simulink model "slGTC_3gdl"  (Simulink 9.0)
settings: Solver=ode45  StartTime=0.0  StopTime=Tsim  MaxStep=1e-3  RelTol=1e-8  EnableMultiTasking=on
values from neighbouring files (symbols this model uses):
  duracion = 1    [simulaciones.m]
  n = 5    [simulaciones.m]
  t_ini = 0.5    [simulaciones.m]
  Tm = 0.001    [Controlre.m]    (also in controles.m; simulaciones.m)
  XYZfin = CinematicaDirecta([1 1 1])    [simulaciones.m]
  XYZini = CinematicaDirecta([0 0 0])    [simulaciones.m]
settings Model: Creator=Manuel G. Ortega  LastModifiedBy=Alvaro  ExtModeTrigMode=oneshot  ExtModeArmWhenConnect=off
settings DataIOCC: SignalLoggingSaveFormat=ModelDataLogs
settings OptimizationCC: BooleanDataType=off  ExpressionDepthLimit=2147483647  InitFltsAndDblsToZero=on
settings DebuggingCC: SaveWithParameterizedLinksMsg=none  SignalResolutionControl=TryResolveAllWithWarning  MultiTaskDSMMsg=warning  MultiTaskCondExecSysMsg=none  FcnCallInpInsideContextMsg=warning  StateNameClashWarn=warning  StrictBusMsg=None
settings HardwareCC: TargetUnknown=on
settings GRTTargetCC: TargetFcnLib=ansi_tfl_tmw.mat  GeneratePreprocessorConditionals=Disable all  CombineOutputUpdateFcns=off  GRTInterface=on
settings ConfigComp: CovSFcnEnable=off

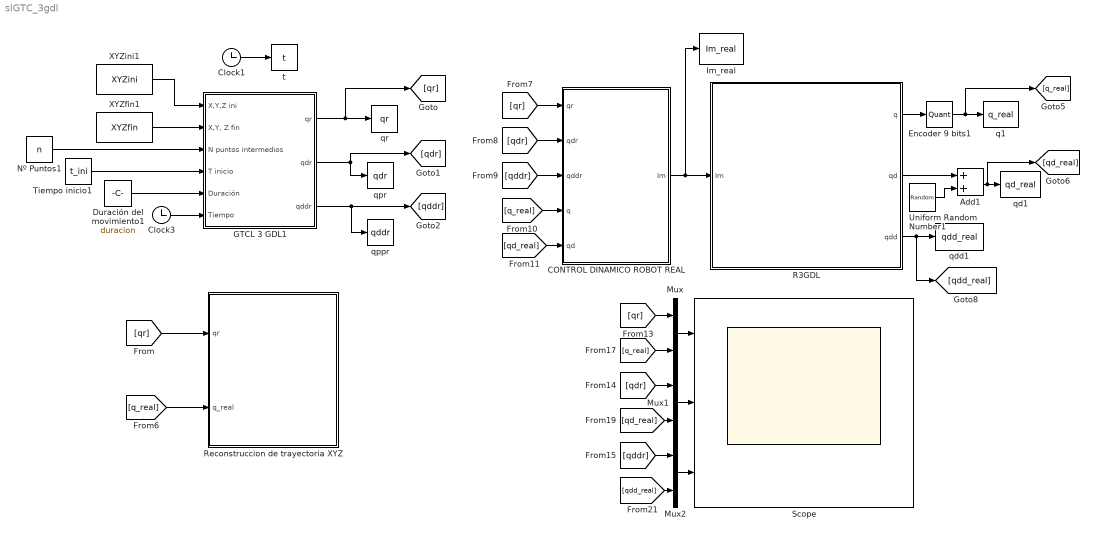
== system slGTC_3gdl ==
  Add1 : Sum
  CONTROL DINAMICO ROBOT REAL : Subsystem
  Clock1 : Clock
  Clock3 : Clock
  Duración del movimiento1 : Constant  Value=duracion
  Encoder 9 bits1 : Quantizer  QuantizationInterval=2*pi/(2^9)
  GTCL 3 GDL1 : Subsystem
  Im_real : ToWorkspace  VariableName=Im_real
  Mux : Mux  Inputs=2
  Mux1 : Mux  Inputs=2
  Mux2 : Mux  Inputs=2
  Nº Puntos1 : Constant  Value=n
  R3GDL : Subsystem  mask(Control y Programación de Robots (4 GIERM)){NGrupo=3, q1_ini=0, q2_ini=0, q3_ini=0, Bl_q1=off, Bl_q2=off, Bl_q3=off, AccionamientoDirecto=on}
      mask prompts: NGrupo "Nº de GRUPO"; q1_ini "q1 inicial  (rad)"; q2_ini "q2 inicial (rad)"; q3_ini "q3_inicial (rad)"; Bl_q1 "Bloqueo q1"; Bl_q2 "Bloqueo q2"; Bl_q3 "Bloqueo q3"; AccionamientoDirecto "Accionamiento directo"
      mask help: Robot de 3 grados de libertad RRR
      mask Display:
      | image(imread('R3GDL_RRR.JPG'));
      | port_label('output', 1, 'q');
      | port_label('output', 2, 'qd');
      | port_label('output', 3, 'qdd');
      | port_label('input', 1, 'Im')
  Reconstruccion de trayectoria XYZ : Subsystem
  Scope : Scope  NumInputPorts=3
  Tiempo inicio1 : Constant  Value=t_ini
  Uniform Random Number1 : UniformRandomNumber  Minimum=-1500*2*pi/60*0.01  Maximum=1500*2*pi/60*0.01  SampleTime=Tm/10
  XYZfin1 : Constant  Value=XYZfin
  XYZini1 : Constant  Value=XYZini
  q1 : ToWorkspace  VariableName=q_real  SampleTime=-1
  qd1 : ToWorkspace  VariableName=qd_real  SampleTime=-1
  qdd1 : ToWorkspace  VariableName=qdd_real  SampleTime=-1
  qppr : ToWorkspace  VariableName=qddr  SampleTime=-1
  qpr : ToWorkspace  VariableName=qdr  SampleTime=-1
  qr : ToWorkspace  VariableName=qr  SampleTime=-1
  t : ToWorkspace  VariableName=t  SampleTime=-1
  wires:
  GTCL 3 GDL1/1(qr) -> [qr], qr/1
  GTCL 3 GDL1/2(qdr) -> qpr/1, [qdr]
  GTCL 3 GDL1/3(qddr) -> qppr/1, [qddr]
  Clock3/1 -> GTCL 3 GDL1/6(Tiempo)
  XYZini1/1 -> GTCL 3 GDL1/1(X,Y,Z ini)
  Clock1/1 -> t/1
  Nº Puntos1/1 -> GTCL 3 GDL1/3(N puntos intermedios)
  Tiempo inicio1/1 -> GTCL 3 GDL1/4(T inicio)
  Duración del movimiento1/1 -> GTCL 3 GDL1/5(Duración)
  XYZfin1/1 -> GTCL 3 GDL1/2("X,Y, Z fin")
  [qd_real] -> CONTROL DINAMICO ROBOT REAL/5(qd)
  [q_real] -> CONTROL DINAMICO ROBOT REAL/4(q)
  [qddr] -> CONTROL DINAMICO ROBOT REAL/3(qddr)
  [qdr] -> CONTROL DINAMICO ROBOT REAL/2(qdr)
  [qr] -> CONTROL DINAMICO ROBOT REAL/1(qr)
  CONTROL DINAMICO ROBOT REAL/1(Im) -> Im_real/1, R3GDL/1(Im)
  R3GDL/3(qdd) -> [qdd_real], qdd1/1
  [qr] -> Reconstruccion de trayectoria XYZ/1(qr)
  [q_real] -> Reconstruccion de trayectoria XYZ/2(q_real)
  Mux/1 -> Scope/1
  Mux1/1 -> Scope/2
  Mux2/1 -> Scope/3
  [qr] -> Mux/1
  [qdr] -> Mux1/1
  [qddr] -> Mux2/1
  [q_real] -> Mux/2
  [qd_real] -> Mux1/2
  [qdd_real] -> Mux2/2
  Uniform Random Number1/1 -> Add1/2
  R3GDL/1(q) -> Encoder 9 bits1/1
  Encoder 9 bits1/1 -> [q_real], q1/1
  R3GDL/2(qd) -> Add1/1
  Add1/1 -> [qd_real], qd1/1

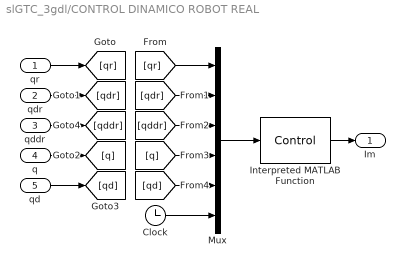
== system slGTC_3gdl/CONTROL DINAMICO ROBOT REAL ==
  qr : Inport
  qdr : Inport  Port=2
  qddr : Inport  Port=3
  q : Inport  Port=4
  qd : Inport  Port=5
  Clock : Clock
  Interpreted MATLAB Function : MATLABFcn  MATLABFcn=Control  SampleTime=Tm
  Mux : Mux  Inputs=6
  Im : Outport
  wires:
  [qddr] -> Mux/3
  [qd] -> Mux/5
  [q] -> Mux/4
  [qr] -> Mux/1
  [qdr] -> Mux/2
  Clock/1 -> Mux/6
  Mux/1 -> Interpreted MATLAB Function/1
  Interpreted MATLAB Function/1 -> Im/1
  qddr/1 -> [qddr]
  qd/1 -> [qd]
  q/1 -> [q]
  qdr/1 -> [qdr]
  qr/1 -> [qr]

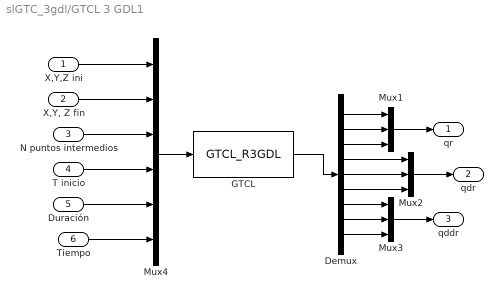
== system slGTC_3gdl/GTCL 3 GDL1 ==
  X,Y,Z ini : Inport
  "X,Y, Z fin" : Inport  Port=2
  N puntos intermedios : Inport  Port=3
  T inicio : Inport  Port=4
  Duración : Inport  Port=5
  Tiempo : Inport  Port=6
  Demux : Demux  Outputs=9
  GTCL : MATLABFcn  MATLABFcn=GTCL_R3GDL  OutputDimensions=9
  Mux1 : Mux  Inputs=3
  Mux2 : Mux  Inputs=3
  Mux3 : Mux  Inputs=3
  Mux4 : Mux  Inputs=6
  qr : Outport
  qdr : Outport  Port=2
  qddr : Outport  Port=3
  wires:
  Mux1/1 -> qr/1
  Mux4/1 -> GTCL/1
  X,Y,Z ini/1 -> Mux4/1
  "X,Y, Z fin"/1 -> Mux4/2
  N puntos intermedios/1 -> Mux4/3
  T inicio/1 -> Mux4/4
  Duración/1 -> Mux4/5
  Tiempo/1 -> Mux4/6
  GTCL/1 -> Demux/1
  Demux/1 -> Mux1/1
  Demux/2 -> Mux1/2
  Demux/3 -> Mux1/3
  Mux2/1 -> qdr/1
  Demux/4 -> Mux2/1
  Demux/5 -> Mux2/2
  Demux/6 -> Mux2/3
  Mux3/1 -> qddr/1
  Demux/7 -> Mux3/1
  Demux/8 -> Mux3/2
  Demux/9 -> Mux3/3

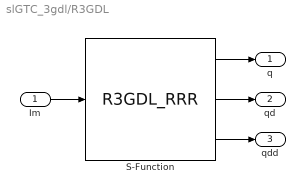
== system slGTC_3gdl/R3GDL ==
  Im : Inport
  S-Function : S-Function  FunctionName=R3GDL_RRR  Parameters=[q1_ini; q2_ini; q3_ini]; [Bl_q1; Bl_q2; Bl_q3]; AccionamientoDirecto; NGrupo  SFunctionDeploymentMode=off  EnableBusSupport=off
  q : Outport
  qd : Outport  Port=2
  qdd : Outport  Port=3
  wires:
  Im/1 -> S-Function/1
  S-Function/1 -> q/1
  S-Function/2 -> qd/1
  S-Function/3 -> qdd/1

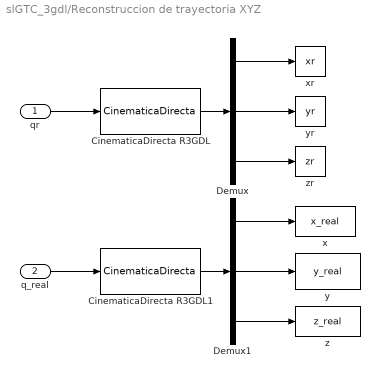
== system slGTC_3gdl/Reconstruccion de trayectoria XYZ ==
  qr : Inport
  q_real : Inport  Port=2
  CinematicaDirecta R3GDL : MATLABFcn  MATLABFcn=CinematicaDirecta
  CinematicaDirecta R3GDL1 : MATLABFcn  MATLABFcn=CinematicaDirecta
  Demux : Demux  Outputs=3
  Demux1 : Demux  Outputs=3
  x : ToWorkspace  VariableName=x_real  SampleTime=-1
  xr : ToWorkspace  VariableName=xr  SampleTime=-1
  y : ToWorkspace  VariableName=y_real  SampleTime=-1
  yr : ToWorkspace  VariableName=yr  SampleTime=-1
  z : ToWorkspace  VariableName=z_real  SampleTime=-1
  zr : ToWorkspace  VariableName=zr  SampleTime=-1
  wires:
  Demux/1 -> xr/1
  CinematicaDirecta R3GDL/1 -> Demux/1
  Demux/2 -> yr/1
  Demux1/1 -> x/1
  Demux/3 -> zr/1
  Demux1/3 -> z/1
  Demux1/2 -> y/1
  CinematicaDirecta R3GDL1/1 -> Demux1/1
  qr/1 -> CinematicaDirecta R3GDL/1
  q_real/1 -> CinematicaDirecta R3GDL1/1
